simulink model "subsistema"  (Simulink 7.7)
settings: Solver=ode45  StartTime=0.0  StopTime=10.0  RelTol=1e-3
settings Model: Creator=George  LastModifiedBy=George

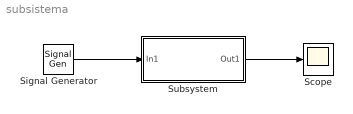
== system subsistema ==
  Scope : Scope
  Signal Generator : SignalGenerator
  Subsystem : Subsystem
  wires:
  Signal Generator/1 -> Subsystem/1(In1)
  Subsystem/1(Out1) -> Scope/1

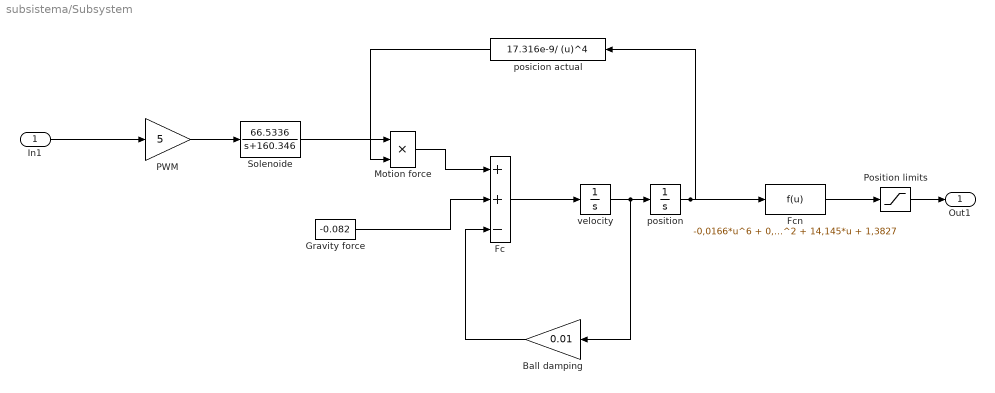
== system subsistema/Subsystem ==
  In1 : Inport
  Ball damping : Gain  Gain=0.01  SaturateOnIntegerOverflow=on  OutDataTypeStr=Inherit: Same as input  ParamDataTypeStr=Inherit: Same as input
  Fc : Sum  Inputs=++-  SaturateOnIntegerOverflow=on  InputSameDT=on  OutDataTypeStr=Inherit: Same as first input
  Fcn : Fcn  Expr=-0,0166*u^6 + 0,3252*u^5 - 2,5048*u^4 + 9,507*u^3 - 17,977*u^2 + 14,145*u + 1,3827
  Gravity force : Constant  Value=-0.082
  Motion force : Product  SaturateOnIntegerOverflow=on  InputSameDT=on  OutDataTypeStr=Inherit: Same as first input
  PWM : Gain  Gain=5  SaturateOnIntegerOverflow=on  OutDataTypeStr=Inherit: Same as input  ParamDataTypeStr=Inherit: Same as input
  Position limits : Saturate  UpperLimit=5  LowerLimit=-5  ZeroCross=off
  Solenoide : TransferFcn  Numerator=[66.5336]  Denominator=[1 160.346]
  posicion actual : Fcn  Expr=17.316e-9/ (u)^4
  position : Integrator  LimitOutput=on  UpperSaturationLimit=0.06  LowerSaturationLimit=0  ZeroCross=off
  velocity : Integrator  UpperSaturationLimit=Inf  LowerSaturationLimit=-Inf  ZeroCross=off
  Out1 : Outport
  wires:
  PWM/1 -> Solenoide/1
  Solenoide/1 -> Motion force/1
  Gravity force/1 -> Fc/2
  Motion force/1 -> Fc/1
  velocity/1 -> position/1, Ball damping/1
  Fc/1 -> velocity/1
  position/1 -> posicion actual/1, Fcn/1
  Ball damping/1 -> Fc/3
  posicion actual/1 -> Motion force/2
  Fcn/1 -> Position limits/1
  In1/1 -> PWM/1
  Position limits/1 -> Out1/1
